simulink model "ES200A_CurrMeas"  (R2013b)
settings: Solver=FixedStepDiscrete  SolverMode=SingleTasking  StartTime=0.0  StopTime=1  FixedStep=0.000125  RelTol=1e-3
values from neighbouring files (symbols this model uses):
  ARCHGLBPRM_2PI_ULS_F32 = DataDict.Constant    [ES200A_CurrMeas_DataDict.m]
  CurrMeasEolGainMax = DataDict.Calibration    [ES200A_CurrMeas_DataDict.m]
  CurrMeasEolGainMin = DataDict.Calibration    [ES200A_CurrMeas_DataDict.m]
  CurrMeasEolGainNrOfSample = DataDict.Calibration    [ES200A_CurrMeas_DataDict.m]
  CurrMeasEolGainNumer = DataDict.Calibration    [ES200A_CurrMeas_DataDict.m]
  CurrMeasEolMaxMotVel = DataDict.Calibration    [ES200A_CurrMeas_DataDict.m]
  CurrMeasEolOffsHiBrdgVltgMin = DataDict.Calibration    [ES200A_CurrMeas_DataDict.m]
  CurrMeasEolOffsHiCmuOffs = DataDict.Calibration    [ES200A_CurrMeas_DataDict.m]
  CurrMeasEolOffsLoCmuOffs = DataDict.Calibration    [ES200A_CurrMeas_DataDict.m]
  CurrMeasEolOffsMax = DataDict.Calibration    [ES200A_CurrMeas_DataDict.m]
  CurrMeasEolOffsMin = DataDict.Calibration    [ES200A_CurrMeas_DataDict.m]
  CurrMeasEolOffsNrOfSample = DataDict.Calibration    [ES200A_CurrMeas_DataDict.m]
  CurrMeasEolTranCntrThd = DataDict.Calibration    [ES200A_CurrMeas_DataDict.m]
  CurrMeasMinRqrdPhaOnTi = DataDict.Calibration    [ES200A_CurrMeas_DataDict.m]
  CurrMeasMotAgCompuDly = DataDict.Calibration    [ES200A_CurrMeas_DataDict.m]
  CurrMeasMotCurrAdcVlyWrmIninMax = DataDict.Calibration    [ES200A_CurrMeas_DataDict.m]
  CurrMeasMotCurrAdcVlyWrmIninMin = DataDict.Calibration    [ES200A_CurrMeas_DataDict.m]
  CurrMeasNtc0x05DFailStep = DataDict.Calibration    [ES200A_CurrMeas_DataDict.m]
  CurrMeasNtc0x05DPassStep = DataDict.Calibration    [ES200A_CurrMeas_DataDict.m]
  CurrMeasNtc0x06DFailStep = DataDict.Calibration    [ES200A_CurrMeas_DataDict.m]
  CurrMeasNtc0x06DPassStep = DataDict.Calibration    [ES200A_CurrMeas_DataDict.m]
  DEGREES30_MOTRAD_F32 = DataDict.Constant    [ES200A_CurrMeas_DataDict.m]
  DIFOFFSRNGCHKMAX_VOLT_F32 = DataDict.Constant    [ES200A_CurrMeas_DataDict.m]
  ELECGLBPRM_IVTRCNT_CNT_U08 = DataDict.ConfigParam    [ES200A_CurrMeas_DataDict.m]
  ELECGLBPRM_STRTUPSTCURRMEASWRMININTESTSTRT_CNT_U08 = DataDict.Constant    [ES200A_CurrMeas_DataDict.m]
  FLTINJ_CURRMEAS_MOTCURRCORRDA = DataDict.Constant    [ES200A_CurrMeas_DataDict.m]
  FLTINJ_CURRMEAS_MOTCURRCORRDD = DataDict.Constant    [ES200A_CurrMeas_DataDict.m]
  FLTINJ_CURRMEAS_TESTOK = DataDict.Constant    [ES200A_CurrMeas_DataDict.m]
  MAXCURRCORRD_AMPR_F32 = DataDict.Constant    [ES200A_CurrMeas_DataDict.m]
  PhaABCMeasdOutOfRng = DataDict.NTC    [ES200A_CurrMeas_DataDict.m]
  PhaDEFMeasOutOfRng = DataDict.NTC    [ES200A_CurrMeas_DataDict.m]
  SysGlbPrmMotPoleCnt = DataDict.ImprtdCal    [ES200A_CurrMeas_DataDict.m]
libraries: simulink x10, FixdToFloat x1
(part 6 of 7)

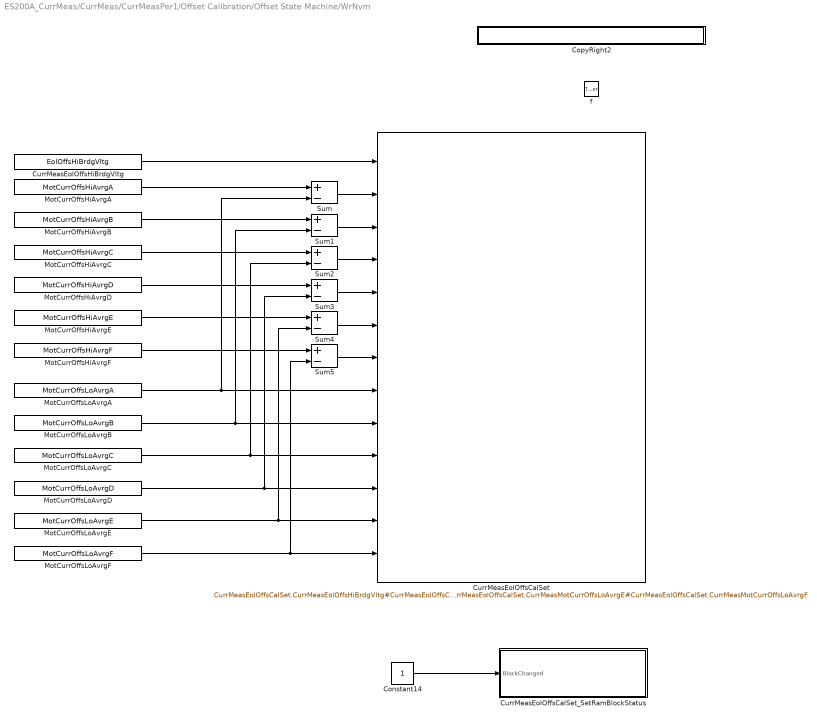
== system ES200A_CurrMeas/CurrMeas/CurrMeasPer1/Offset Calibration/Offset State Machine/WrNvm ==
  f : TriggerPort  TriggerType=function-call
      settings: CopyFcn=Stateflow.SLINSF.SimulinkMan.removeBlockPreDeleteFcn  PreDeleteFcn=Stateflow.SLINSF.SimulinkMan.unsafePredeleteFcn
  Constant14 : Constant  OutDataTypeStr=single
  CopyRight2 : Subsystem  Description=|  mask(Copyright Information){none=on}
      | Copyright info block.                                               
      |                                                                     
      | Place copyright information at the top of every subsystem in design.
      mask prompts: none "No parameters"
      mask help: Place copyright information at the top of every subsystem in design.
      mask Display:
      | NxtrConf = 'Nexteer Confidential';
      | 
      | sys = bdroot; %handle for the current model ("system")
      | first = get_param(sys,'Created');
      | first = first(end-3:end);  %year is last four digits
      | 
      | last = get_param(sys,'LastModifiedDate');
      | if isempty(last)
      |     last = datestr(now,'yyyy');
      | else
      |     last = last(end-3:end);
      | end
      | 
      | if strcmp(first,last)
      |     fprintf('%s -- Copyright %s Nexteer',NxtrConf,first)
      | else
      |     fprintf('%s -- %s%s- %s Nexteer',NxtrConf,char(169),first,last)
      | end
  CurrMeasEolOffsCalSet : DataStoreWrite  RequirementInfo={'linktype_rmi_doors' '000089bc (/ESG Group/FDD Module Requirements/EA4 Specific/ES200A_CurrMeas)' '#ES200A_138' 'true' 'REQ: ES200A_138' '' } %GIDa_9629138e_22c6_4a2f_a212_b03a049f0344  DataStoreName=CurrMeasEolOffsCalSet  DataStoreElements=CurrMeasEolOffsCalSet.CurrMeasEolOffsHiBrdgVltg#CurrMeasEolOffsCalSet.CurrMeasMotCurrEolOffsDifA#CurrMeasEolOffsCalSet.CurrMeasMotCurrEolOffsDifB#CurrMeasEolOffsCalSet.CurrMeasMotCurrEolOffsDifC#CurrMeasEolOffsCalSet.CurrMeasMotCurrEolOffsDifD#CurrMeasEolOffsCalSet.CurrMeasMotCurrEolOffsDifE#CurrMeasEolOffsCalSet.CurrMeasMotCurrEolOffsDifF#CurrMeasEolOffsCalSet.CurrMeasMotCurrOffsLoAvrgA#CurrMeasEolOffsCalSet.CurrMeasMotCurrOffsLoAvrgB#CurrMeasEolOffsCalSet.CurrMeasMotCurrOffsLoAvrgC#CurrMeasEolOffsCalSet.CurrMeasMotCurrOffsLoAvrgD#CurrMeasEolOffsCalSet.CurrMeasMotCurrOffsLoAvrgE#CurrMeasEolOffsCalSet.CurrMeasMotCurrOffsLoAvrgF
  CurrMeasEolOffsCalSet_SetRamBlockStatus : Subsystem  RequirementInfo={'linktype_rmi_doors' '000089bc (/ESG Group/FDD Module Requirements/EA4 Specific/ES200A_CurrMeas)' '#ES200A_138' 'true' 'REQ: ES200A_138' '' } %GIDa_8abdf95c_ca53_47b3_a6c5_ea06d33b5ee8  TreatAsAtomicUnit=on
  CurrMeasEolOffsHiBrdgVltg : DataStoreRead  DataStoreName=EolOffsHiBrdgVltg  DataStoreElements=EolOffsHiBrdgVltg
  MotCurrOffsHiAvrgA : DataStoreRead  DataStoreName=MotCurrOffsHiAvrgA  DataStoreElements=MotCurrOffsHiAvrgA
  MotCurrOffsHiAvrgB : DataStoreRead  DataStoreName=MotCurrOffsHiAvrgB  DataStoreElements=MotCurrOffsHiAvrgB
  MotCurrOffsHiAvrgC : DataStoreRead  DataStoreName=MotCurrOffsHiAvrgC  DataStoreElements=MotCurrOffsHiAvrgC
  MotCurrOffsHiAvrgD : DataStoreRead  DataStoreName=MotCurrOffsHiAvrgD  DataStoreElements=MotCurrOffsHiAvrgD
  MotCurrOffsHiAvrgE : DataStoreRead  DataStoreName=MotCurrOffsHiAvrgE  DataStoreElements=MotCurrOffsHiAvrgE
  MotCurrOffsHiAvrgF : DataStoreRead  DataStoreName=MotCurrOffsHiAvrgF  DataStoreElements=MotCurrOffsHiAvrgF
  MotCurrOffsLoAvrgA : DataStoreRead  DataStoreName=MotCurrOffsLoAvrgA  DataStoreElements=MotCurrOffsLoAvrgA
  MotCurrOffsLoAvrgB : DataStoreRead  DataStoreName=MotCurrOffsLoAvrgB  DataStoreElements=MotCurrOffsLoAvrgB
  MotCurrOffsLoAvrgC : DataStoreRead  DataStoreName=MotCurrOffsLoAvrgC  DataStoreElements=MotCurrOffsLoAvrgC
  MotCurrOffsLoAvrgD : DataStoreRead  DataStoreName=MotCurrOffsLoAvrgD  DataStoreElements=MotCurrOffsLoAvrgD
  MotCurrOffsLoAvrgE : DataStoreRead  DataStoreName=MotCurrOffsLoAvrgE  DataStoreElements=MotCurrOffsLoAvrgE
  MotCurrOffsLoAvrgF : DataStoreRead  DataStoreName=MotCurrOffsLoAvrgF  DataStoreElements=MotCurrOffsLoAvrgF
  Sum{,1..5} (6 alike) : Sum  Inputs=+-
  wires:
  CurrMeasEolOffsHiBrdgVltg/1 -> CurrMeasEolOffsCalSet/1
  Sum/1 -> CurrMeasEolOffsCalSet/2
  Sum1/1 -> CurrMeasEolOffsCalSet/3
  Sum2/1 -> CurrMeasEolOffsCalSet/4
  Sum3/1 -> CurrMeasEolOffsCalSet/5
  Sum4/1 -> CurrMeasEolOffsCalSet/6
  Sum5/1 -> CurrMeasEolOffsCalSet/7
  MotCurrOffsLoAvrgC/1 -> Sum2/2, CurrMeasEolOffsCalSet/10
  MotCurrOffsLoAvrgB/1 -> Sum1/2, CurrMeasEolOffsCalSet/9
  MotCurrOffsLoAvrgD/1 -> Sum3/2, CurrMeasEolOffsCalSet/11
  MotCurrOffsLoAvrgE/1 -> Sum4/2, CurrMeasEolOffsCalSet/12
  MotCurrOffsLoAvrgA/1 -> Sum/2, CurrMeasEolOffsCalSet/8
  MotCurrOffsLoAvrgF/1 -> CurrMeasEolOffsCalSet/13, Sum5/2
  Constant14/1 -> CurrMeasEolOffsCalSet_SetRamBlockStatus/1("BlockChanged ")
  MotCurrOffsHiAvrgA/1 -> Sum/1
  MotCurrOffsHiAvrgB/1 -> Sum1/1
  MotCurrOffsHiAvrgC/1 -> Sum2/1
  MotCurrOffsHiAvrgD/1 -> Sum3/1
  MotCurrOffsHiAvrgE/1 -> Sum4/1
  MotCurrOffsHiAvrgF/1 -> Sum5/1

== system ES200A_CurrMeas/CurrMeas/CurrMeasPer2/Chart1/CalcMotCurrMotAgCorrd/+//- 2*Pi Rollover ==
  MotAgCorrdRaw : Inport
  -2*pi Rollover : Subsystem  TreatAsAtomicUnit=on
  2*pi Rollover : Subsystem  TreatAsAtomicUnit=on
  Constant : Constant  Value=-1  OutDataTypeStr=single
  Constant1 : Constant  Value=ARCHGLBPRM_2PI_ULS_F32  OutDataTypeStr=Inherit: Inherit via back propagation
  Constant4 : Constant  Value=ARCHGLBPRM_2PI_ULS_F32  OutDataTypeStr=Inherit: Inherit via back propagation
  CopyRight2 : Subsystem  Description=|  mask(Copyright Information){none=on}
      | Copyright info block.                                               
      |                                                                     
      | Place copyright information at the top of every subsystem in design.
      mask prompts: none "No parameters"
      mask help: Place copyright information at the top of every subsystem in design.
      mask Display:
      | NxtrConf = 'Nexteer Confidential';
      | 
      | sys = bdroot; %handle for the current model ("system")
      | first = get_param(sys,'Created');
      | first = first(end-3:end);  %year is last four digits
      | 
      | last = get_param(sys,'LastModifiedDate');
      | if isempty(last)
      |     last = datestr(now,'yyyy');
      | else
      |     last = last(end-3:end);
      | end
      | 
      | if strcmp(first,last)
      |     fprintf('%s -- Copyright %s Nexteer',NxtrConf,first)
      | else
      |     fprintf('%s -- %s%s- %s Nexteer',NxtrConf,char(169),first,last)
      | end
  If : If  NumInputs=3  IfExpression=u1 > u2  ElseIfExpressions=u1 < u3
  Merge : Merge  Inputs=3
  Pass Through : Subsystem  TreatAsAtomicUnit=on
  Product : Product
  MotCtrlCurrMeasMotAgCorrd : Outport
  wires:
  If/2 -> -2*pi Rollover/Action
  MotAgCorrdRaw/1 -> If/1, [MotAgCorrdRaw]
  Constant4/1 -> If/2
  Constant1/1 -> Product/1
  If/1 -> 2*pi Rollover/Action
  [MotAgCorrdRaw] -> 2*pi Rollover/1(MotAgCorrdRaw)
  [MotAgCorrdRaw] -> -2*pi Rollover/1(MotAgCorrdRaw)
  If/3 -> Pass Through/Action
  2*pi Rollover/1(Out1) -> Merge/1
  -2*pi Rollover/1(Out1) -> Merge/2
  Pass Through/1(Out1) -> Merge/3
  [MotAgCorrdRaw] -> Pass Through/1(MotAgCorrdRaw)
  Merge/1 -> MotCtrlCurrMeasMotAgCorrd/1
  Constant/1 -> Product/2
  Product/1 -> If/3

== system ES200A_CurrMeas/CurrMeas/CurrMeasPer2/Chart1/CalcMotCurrMotAgCorrd/CopyRight2 ==

== system ES200A_CurrMeas/CurrMeas/CurrMeasPer2/Chart1/OffsCalcABC/CopyRight2 ==

== system ES200A_CurrMeas/CurrMeas/CurrMeasPer2/Chart1/OffsCalcDEF/CopyRight2 ==

== system ES200A_CurrMeas/CurrMeas/CurrMeasPer2/Chart1/ProtocolChkENABC/CopyRight2 ==

== system ES200A_CurrMeas/CurrMeas/CurrMeasPer2/Chart1/ProtocolChkENABC/FltInj_u08 ==
  note: This block requires no modification by FDD author.
      |
      | This block does not actually simulate any fault injection.  It is simply a pass-thru.
      |
      | The Constant port (#2) simply terminates its signal, but we are trying to force the FDD author
      | to properly use the FltInjectionLocType enumeration in FDD model.
  note: EA4.x Fault Injection
  Signal_In : Inport
  Constant : Inport  Port=2
  CopyRight2 : Subsystem  Description=|  mask(Copyright Information){none=on}
      | Copyright info block.                                               
      |                                                                     
      | Place copyright information at the top of every subsystem in design.
      mask prompts: none "No parameters"
      mask help: Place copyright information at the top of every subsystem in design.
      mask Display:
      | NxtrConf = 'Nexteer Confidential';
      | 
      | sys = bdroot; %handle for the current model ("system")
      | first = get_param(sys,'Created');
      | first = first(end-3:end);  %year is last four digits
      | 
      | last = get_param(sys,'LastModifiedDate');
      | if isempty(last)
      |     last = datestr(now,'yyyy');
      | else
      |     last = last(end-3:end);
      | end
      | 
      | if strcmp(first,last)
      |     fprintf('%s -- Copyright %s Nexteer',NxtrConf,first)
      | else
      |     fprintf('%s -- %s%s- %s Nexteer',NxtrConf,char(169),first,last)
      | end
  Terminator : Terminator
  Signal_Out : Outport
  wires:
  Signal_In/1 -> Signal_Out/1
  Constant/1 -> Terminator/1

== system ES200A_CurrMeas/CurrMeas/CurrMeasPer2/Chart1/ProtocolChkENDEF/CopyRight2 ==

== system ES200A_CurrMeas/CurrMeas/CurrMeasPer2/FltInj_f32/CopyRight2 ==

== system ES200A_CurrMeas/CurrMeas/CurrMeasPer3/Chart1/GetNtc5DQlfrSts/CopyRight2 ==

== system ES200A_CurrMeas/CurrMeas/CurrMeasPer3/Chart1/GetNtc5DQlfrSts/GetNtcQlfrSts ==
  NtcNr : Inport
  CopyRight2 : Subsystem  Description=|  mask(Copyright Information){none=on}
      | Copyright info block.                                               
      |                                                                     
      | Place copyright information at the top of every subsystem in design.
      mask prompts: none "No parameters"
      mask help: Place copyright information at the top of every subsystem in design.
      mask Display:
      | NxtrConf = 'Nexteer Confidential';
      | 
      | sys = bdroot; %handle for the current model ("system")
      | first = get_param(sys,'Created');
      | first = first(end-3:end);  %year is last four digits
      | 
      | last = get_param(sys,'LastModifiedDate');
      | if isempty(last)
      |     last = datestr(now,'yyyy');
      | else
      |     last = last(end-3:end);
      | end
      | 
      | if strcmp(first,last)
      |     fprintf('%s -- Copyright %s Nexteer',NxtrConf,first)
      | else
      |     fprintf('%s -- %s%s- %s Nexteer',NxtrConf,char(169),first,last)
      | end
  Data Store Read1 : DataStoreRead  DataStoreName=NtcQlfr5D
  Terminator1 : Terminator
  NtcQlfr : Outport
  wires:
  NtcNr/1 -> Terminator1/1
  Data Store Read1/1 -> NtcQlfr/1

== system ES200A_CurrMeas/CurrMeas/CurrMeasPer3/Chart1/GetNtc6DQlfrSts/CopyRight2 ==

== system ES200A_CurrMeas/CurrMeas/CurrMeasPer3/Chart1/GetNtc6DQlfrSts/GetNtcQlfrSts ==
  NtcNr : Inport
  CopyRight2 : Subsystem  Description=|  mask(Copyright Information){none=on}
      | Copyright info block.                                               
      |                                                                     
      | Place copyright information at the top of every subsystem in design.
      mask prompts: none "No parameters"
      mask help: Place copyright information at the top of every subsystem in design.
      mask Display:
      | NxtrConf = 'Nexteer Confidential';
      | 
      | sys = bdroot; %handle for the current model ("system")
      | first = get_param(sys,'Created');
      | first = first(end-3:end);  %year is last four digits
      | 
      | last = get_param(sys,'LastModifiedDate');
      | if isempty(last)
      |     last = datestr(now,'yyyy');
      | else
      |     last = last(end-3:end);
      | end
      | 
      | if strcmp(first,last)
      |     fprintf('%s -- Copyright %s Nexteer',NxtrConf,first)
      | else
      |     fprintf('%s -- %s%s- %s Nexteer',NxtrConf,char(169),first,last)
      | end
  Data Store Read2 : DataStoreRead  DataStoreName=NtcQlfr6D
  Terminator1 : Terminator
  NtcQlfr : Outport
  wires:
  NtcNr/1 -> Terminator1/1
  Data Store Read2/1 -> NtcQlfr/1

== system ES200A_CurrMeas/CurrMeas/CurrMeasPer3/Chart1/RangeChkWIABC/CopyRight2 ==

== system ES200A_CurrMeas/CurrMeas/CurrMeasPer3/Chart1/RangeChkWIABC/If Action Subsystem2 ==
  Action Port : ActionPort  ActionType=then
  Constant : Constant
  CopyRight2 : Subsystem  Description=|  mask(Copyright Information){none=on}
      | Copyright info block.                                               
      |                                                                     
      | Place copyright information at the top of every subsystem in design.
      mask prompts: none "No parameters"
      mask help: Place copyright information at the top of every subsystem in design.
      mask Display:
      | NxtrConf = 'Nexteer Confidential';
      | 
      | sys = bdroot; %handle for the current model ("system")
      | first = get_param(sys,'Created');
      | first = first(end-3:end);  %year is last four digits
      | 
      | last = get_param(sys,'LastModifiedDate');
      | if isempty(last)
      |     last = datestr(now,'yyyy');
      | else
      |     last = last(end-3:end);
      | end
      | 
      | if strcmp(first,last)
      |     fprintf('%s -- Copyright %s Nexteer',NxtrConf,first)
      | else
      |     fprintf('%s -- %s%s- %s Nexteer',NxtrConf,char(169),first,last)
      | end
  Out1 : Outport
  wires:
  Constant/1 -> Out1/1

== system ES200A_CurrMeas/CurrMeas/CurrMeasPer3/Chart1/RangeChkWIABC/If Action Subsystem3 ==
  Action Port : ActionPort  ActionType=else
  Constant : Constant  Value=0
  CopyRight2 : Subsystem  Description=|  mask(Copyright Information){none=on}
      | Copyright info block.                                               
      |                                                                     
      | Place copyright information at the top of every subsystem in design.
      mask prompts: none "No parameters"
      mask help: Place copyright information at the top of every subsystem in design.
      mask Display:
      | NxtrConf = 'Nexteer Confidential';
      | 
      | sys = bdroot; %handle for the current model ("system")
      | first = get_param(sys,'Created');
      | first = first(end-3:end);  %year is last four digits
      | 
      | last = get_param(sys,'LastModifiedDate');
      | if isempty(last)
      |     last = datestr(now,'yyyy');
      | else
      |     last = last(end-3:end);
      | end
      | 
      | if strcmp(first,last)
      |     fprintf('%s -- Copyright %s Nexteer',NxtrConf,first)
      | else
      |     fprintf('%s -- %s%s- %s Nexteer',NxtrConf,char(169),first,last)
      | end
  Out1 : Outport
  wires:
  Constant/1 -> Out1/1

== system ES200A_CurrMeas/CurrMeas/CurrMeasPer3/Chart1/RangeChkWIDEF/CopyRight2 ==

== system ES200A_CurrMeas/CurrMeas/CurrMeasPer3/Chart1/RangeChkWIDEF/If Action Subsystem2 ==
  Action Port : ActionPort  ActionType=then
  Constant : Constant
  CopyRight2 : Subsystem  Description=|  mask(Copyright Information){none=on}
      | Copyright info block.                                               
      |                                                                     
      | Place copyright information at the top of every subsystem in design.
      mask prompts: none "No parameters"
      mask help: Place copyright information at the top of every subsystem in design.
      mask Display:
      | NxtrConf = 'Nexteer Confidential';
      | 
      | sys = bdroot; %handle for the current model ("system")
      | first = get_param(sys,'Created');
      | first = first(end-3:end);  %year is last four digits
      | 
      | last = get_param(sys,'LastModifiedDate');
      | if isempty(last)
      |     last = datestr(now,'yyyy');
      | else
      |     last = last(end-3:end);
      | end
      | 
      | if strcmp(first,last)
      |     fprintf('%s -- Copyright %s Nexteer',NxtrConf,first)
      | else
      |     fprintf('%s -- %s%s- %s Nexteer',NxtrConf,char(169),first,last)
      | end
  Out1 : Outport
  wires:
  Constant/1 -> Out1/1

== system ES200A_CurrMeas/CurrMeas/CurrMeasPer3/Chart1/RangeChkWIDEF/If Action Subsystem3 ==
  Action Port : ActionPort  ActionType=else
  Constant : Constant  Value=0
  CopyRight2 : Subsystem  Description=|  mask(Copyright Information){none=on}
      | Copyright info block.                                               
      |                                                                     
      | Place copyright information at the top of every subsystem in design.
      mask prompts: none "No parameters"
      mask help: Place copyright information at the top of every subsystem in design.
      mask Display:
      | NxtrConf = 'Nexteer Confidential';
      | 
      | sys = bdroot; %handle for the current model ("system")
      | first = get_param(sys,'Created');
      | first = first(end-3:end);  %year is last four digits
      | 
      | last = get_param(sys,'LastModifiedDate');
      | if isempty(last)
      |     last = datestr(now,'yyyy');
      | else
      |     last = last(end-3:end);
      | end
      | 
      | if strcmp(first,last)
      |     fprintf('%s -- Copyright %s Nexteer',NxtrConf,first)
      | else
      |     fprintf('%s -- %s%s- %s Nexteer',NxtrConf,char(169),first,last)
      | end
  Out1 : Outport
  wires:
  Constant/1 -> Out1/1

== system ES200A_CurrMeas/CurrMeas/CurrMeasPer3/Chart1/SetNtc5DSts/CopyRight2 ==

== system ES200A_CurrMeas/CurrMeas/CurrMeasPer3/Chart1/SetNtc5DSts/SetNtcSts ==
  note: Note:
      |
      | - "ISO Fault Debounce Design" Simulink block intent to use here for Simulation purpose only. Do not Code this block
  note: 1. Moved condition Action {ErrAcc = 0;
      | Qualifier =0;
      | } from 2nd Transition action to first trnasition action as there is no condition action in first transition action
      | Also changed SvcClr to 1
  NtcNr : Inport
  NtcStInfo : Inport  Port=2
  NtcSts : Inport  Port=3
  DebStep : Inport  Port=4
  CopyRight2 : Subsystem  Description=|  mask(Copyright Information){none=on}
      | Copyright info block.                                               
      |                                                                     
      | Place copyright information at the top of every subsystem in design.
      mask prompts: none "No parameters"
      mask help: Place copyright information at the top of every subsystem in design.
      mask Display:
      | NxtrConf = 'Nexteer Confidential';
      | 
      | sys = bdroot; %handle for the current model ("system")
      | first = get_param(sys,'Created');
      | first = first(end-3:end);  %year is last four digits
      | 
      | last = get_param(sys,'LastModifiedDate');
      | if isempty(last)
      |     last = datestr(now,'yyyy');
      | else
      |     last = last(end-3:end);
      | end
      | 
      | if strcmp(first,last)
      |     fprintf('%s -- Copyright %s Nexteer',NxtrConf,first)
      | else
      |     fprintf('%s -- %s%s- %s Nexteer',NxtrConf,char(169),first,last)
      | end
  Data Store Write : DataStoreWrite  DataStoreName=NtcQlfr5D
  Ground : Ground
  ISO Fault Debounce Design : Stateflow chart  TreatAsAtomicUnit=on
      settings: AttributesFormatString=|
      | Simulation Purpose Only.
      | Do Not Code this block
      | Diagnostic Manager Owns this requirement
  Scope1 : Scope  NumInputPorts=3
      settings: YMin=2~16384~-5  YMax=2~16384~5  SaveName=ScopeData5
  Terminator : Terminator
  Terminator1 : Terminator
  wires:
  NtcStInfo/1 -> Terminator1/1
  NtcNr/1 -> Terminator/1
  NtcSts/1 -> ISO Fault Debounce Design/1(NtcSts), Scope1/1
  DebStep/1 -> ISO Fault Debounce Design/2(DebStep), Scope1/2
  ISO Fault Debounce Design/1(Qualifier) -> Data Store Write/1, Scope1/3
  Ground/1 -> ISO Fault Debounce Design/3(SvcClr)

== system ES200A_CurrMeas/CurrMeas/CurrMeasPer3/Chart1/SetNtc6DSts/CopyRight2 ==

== system ES200A_CurrMeas/CurrMeas/CurrMeasPer3/Chart1/SetNtc6DSts/SetNtcSts ==
  note: Note:
      |
      | - "ISO Fault Debounce Design" Simulink block intent to use here for Simulation purpose only. Do not Code this block
  note: Moved condition Action {ErrAcc = 0;
      | Qualifier =0;
      | } from 2nd Transition action to first trnasition action as there is no condition action in first transition action
      | Also changed SvcClr to 1
  NtcNr : Inport
  NtcStInfo : Inport  Port=2
  NtcSts : Inport  Port=3
  DebStep : Inport  Port=4
  CopyRight2 : Subsystem  Description=|  mask(Copyright Information){none=on}
      | Copyright info block.                                               
      |                                                                     
      | Place copyright information at the top of every subsystem in design.
      mask prompts: none "No parameters"
      mask help: Place copyright information at the top of every subsystem in design.
      mask Display:
      | NxtrConf = 'Nexteer Confidential';
      | 
      | sys = bdroot; %handle for the current model ("system")
      | first = get_param(sys,'Created');
      | first = first(end-3:end);  %year is last four digits
      | 
      | last = get_param(sys,'LastModifiedDate');
      | if isempty(last)
      |     last = datestr(now,'yyyy');
      | else
      |     last = last(end-3:end);
      | end
      | 
      | if strcmp(first,last)
      |     fprintf('%s -- Copyright %s Nexteer',NxtrConf,first)
      | else
      |     fprintf('%s -- %s%s- %s Nexteer',NxtrConf,char(169),first,last)
      | end
  Data Store Write : DataStoreWrite  DataStoreName=NtcQlfr6D
  Ground : Ground
  ISO Fault Debounce Design : Stateflow chart  TreatAsAtomicUnit=on
      settings: AttributesFormatString=|
      | Simulation Purpose Only.
      | Do Not Code this block
      | Diagnostic Manager Owns this requirement
  Scope1 : Scope  NumInputPorts=3
      settings: YMin=-5~-5~-5  YMax=5~5~5  SaveName=ScopeData5
  Terminator : Terminator
  Terminator1 : Terminator
  wires:
  NtcStInfo/1 -> Terminator1/1
  NtcNr/1 -> Terminator/1
  NtcSts/1 -> ISO Fault Debounce Design/1(NtcSts), Scope1/1
  DebStep/1 -> ISO Fault Debounce Design/2(DebStep), Scope1/2
  ISO Fault Debounce Design/1(Qualifier) -> Data Store Write/1, Scope1/3
  Ground/1 -> ISO Fault Debounce Design/3(SvcClr)

== system ES200A_CurrMeas/CurrMeas/CurrMeasGainWrReq/IF/CurrMeasEolGainCalSet_SetRamBlockStatus/CopyRight2 ==

== system ES200A_CurrMeas/CurrMeas/CurrMeasOffsWrReq/IF/CurrMeasEolOffsCalSet_SetRamBlockStatus/CopyRight2 ==

== system ES200A_CurrMeas/CurrMeas/CurrMeasPer1/Gain Calibration/GainStateMachine/SetNtcSts/CopyRight2 ==

== system ES200A_CurrMeas/CurrMeas/CurrMeasPer1/Gain Calibration/GainStateMachine/SetNtcSts/SetNtcSts ==
  note: Note:
      |
      | - "ISO Fault Debounce Design" Simulink block intent to use here for Simulation purpose only. Do not Code this block
  NtcNr : Inport
  NtcStInfo : Inport  Port=2
  NtcSts : Inport  Port=3
  DebStep : Inport  Port=4
  CopyRight2 : Subsystem  Description=|  mask(Copyright Information){none=on}
      | Copyright info block.                                               
      |                                                                     
      | Place copyright information at the top of every subsystem in design.
      mask prompts: none "No parameters"
      mask help: Place copyright information at the top of every subsystem in design.
      mask Display:
      | NxtrConf = 'Nexteer Confidential';
      | 
      | sys = bdroot; %handle for the current model ("system")
      | first = get_param(sys,'Created');
      | first = first(end-3:end);  %year is last four digits
      | 
      | last = get_param(sys,'LastModifiedDate');
      | if isempty(last)
      |     last = datestr(now,'yyyy');
      | else
      |     last = last(end-3:end);
      | end
      | 
      | if strcmp(first,last)
      |     fprintf('%s -- Copyright %s Nexteer',NxtrConf,first)
      | else
      |     fprintf('%s -- %s%s- %s Nexteer',NxtrConf,char(169),first,last)
      | end
  Data Store Write : DataStoreWrite  DataStoreName=NtcQlfr1ED
  Ground : Ground
  ISO Fault Debounce Design : Stateflow chart  TreatAsAtomicUnit=on
      settings: AttributesFormatString=|
      | Simulation Purpose Only.
      | Do Not Code this block
      | Diagnostic Manager Owns this requirement
  Scope1 : Scope  NumInputPorts=3
      settings: YMin=-5~-5~-5  YMax=5~5~5  SaveName=ScopeData4
  Terminator : Terminator
  Terminator1 : Terminator
  wires:
  NtcStInfo/1 -> Terminator1/1
  NtcNr/1 -> Terminator/1
  NtcSts/1 -> ISO Fault Debounce Design/1(NtcSts), Scope1/1
  DebStep/1 -> ISO Fault Debounce Design/2(DebStep), Scope1/2
  ISO Fault Debounce Design/1(Qualifier) -> Scope1/3, Data Store Write/1  "Qualifier"
  Ground/1 -> ISO Fault Debounce Design/3(SvcClr)

== system ES200A_CurrMeas/CurrMeas/CurrMeasPer1/Gain Calibration/GainStateMachine/WrNvm/CopyRight2 ==

== system ES200A_CurrMeas/CurrMeas/CurrMeasPer1/Gain Calibration/GainStateMachine/WrNvm/CurrMeasEolGainCalSet_SetRamBlockStatus ==
  "BlockChanged " : Inport  RequirementInfo={} %GIDa_e825a47e_fdb5_416f_b5f2_d196e0b30ed6  OutDataTypeStr=single
  CopyRight2 : Subsystem  Description=|  mask(Copyright Information){none=on}
      | Copyright info block.                                               
      |                                                                     
      | Place copyright information at the top of every subsystem in design.
      mask prompts: none "No parameters"
      mask help: Place copyright information at the top of every subsystem in design.
      mask Display:
      | NxtrConf = 'Nexteer Confidential';
      | 
      | sys = bdroot; %handle for the current model ("system")
      | first = get_param(sys,'Created');
      | first = first(end-3:end);  %year is last four digits
      | 
      | last = get_param(sys,'LastModifiedDate');
      | if isempty(last)
      |     last = datestr(now,'yyyy');
      | else
      |     last = last(end-3:end);
      | end
      | 
      | if strcmp(first,last)
      |     fprintf('%s -- Copyright %s Nexteer',NxtrConf,first)
      | else
      |     fprintf('%s -- %s%s- %s Nexteer',NxtrConf,char(169),first,last)
      | end
  Terminator9 : Terminator
  wires:
  "BlockChanged "/1 -> Terminator9/1

== system ES200A_CurrMeas/CurrMeas/CurrMeasPer1/Offset Calibration/Offset State Machine/SetNtcSts/CopyRight2 ==

== system ES200A_CurrMeas/CurrMeas/CurrMeasPer1/Offset Calibration/Offset State Machine/SetNtcSts/SetNtcSts ==
  note: Note:
      |
      | - "ISO Fault Debounce Design" Simulink block intent to use here for Simulation purpose only. Do not Code this block
  NtcNr : Inport
  NtcStInfo : Inport  Port=2
  NtcSts : Inport  Port=3
  DebStep : Inport  Port=4
  CopyRight2 : Subsystem  Description=|  mask(Copyright Information){none=on}
      | Copyright info block.                                               
      |                                                                     
      | Place copyright information at the top of every subsystem in design.
      mask prompts: none "No parameters"
      mask help: Place copyright information at the top of every subsystem in design.
      mask Display:
      | NxtrConf = 'Nexteer Confidential';
      | 
      | sys = bdroot; %handle for the current model ("system")
      | first = get_param(sys,'Created');
      | first = first(end-3:end);  %year is last four digits
      | 
      | last = get_param(sys,'LastModifiedDate');
      | if isempty(last)
      |     last = datestr(now,'yyyy');
      | else
      |     last = last(end-3:end);
      | end
      | 
      | if strcmp(first,last)
      |     fprintf('%s -- Copyright %s Nexteer',NxtrConf,first)
      | else
      |     fprintf('%s -- %s%s- %s Nexteer',NxtrConf,char(169),first,last)
      | end
  Data Store Write : DataStoreWrite  DataStoreName=NtcQlfr1EC
  Ground : Ground
  ISO Fault Debounce Design : Stateflow chart  TreatAsAtomicUnit=on
      settings: AttributesFormatString=|
      | Simulation Purpose Only.
      | Do Not Code this block
      | Diagnostic Manager Owns this requirement
  Scope1 : Scope  NumInputPorts=3
      settings: YMin=-5~-5~-5  YMax=5~5~5  SaveName=ScopeData4
  Terminator : Terminator
  Terminator1 : Terminator
  wires:
  NtcStInfo/1 -> Terminator1/1
  NtcNr/1 -> Terminator/1
  NtcSts/1 -> ISO Fault Debounce Design/1(NtcSts), Scope1/1
  DebStep/1 -> ISO Fault Debounce Design/2(DebStep), Scope1/2
  ISO Fault Debounce Design/1(Qualifier) -> Scope1/3, Data Store Write/1  "Qualifier"
  Ground/1 -> ISO Fault Debounce Design/3(SvcClr)

== system ES200A_CurrMeas/CurrMeas/CurrMeasPer1/Offset Calibration/Offset State Machine/WrNvm/CopyRight2 ==

== system ES200A_CurrMeas/CurrMeas/CurrMeasPer1/Offset Calibration/Offset State Machine/WrNvm/CurrMeasEolOffsCalSet_SetRamBlockStatus ==
  "BlockChanged " : Inport  RequirementInfo={} %GIDa_ddbbad63_9bf8_4c81_98ef_dae72675538a  OutDataTypeStr=single
  CopyRight2 : Subsystem  Description=|  mask(Copyright Information){none=on}
      | Copyright info block.                                               
      |                                                                     
      | Place copyright information at the top of every subsystem in design.
      mask prompts: none "No parameters"
      mask help: Place copyright information at the top of every subsystem in design.
      mask Display:
      | NxtrConf = 'Nexteer Confidential';
      | 
      | sys = bdroot; %handle for the current model ("system")
      | first = get_param(sys,'Created');
      | first = first(end-3:end);  %year is last four digits
      | 
      | last = get_param(sys,'LastModifiedDate');
      | if isempty(last)
      |     last = datestr(now,'yyyy');
      | else
      |     last = last(end-3:end);
      | end
      | 
      | if strcmp(first,last)
      |     fprintf('%s -- Copyright %s Nexteer',NxtrConf,first)
      | else
      |     fprintf('%s -- %s%s- %s Nexteer',NxtrConf,char(169),first,last)
      | end
  Terminator9 : Terminator
  wires:
  "BlockChanged "/1 -> Terminator9/1

== system ES200A_CurrMeas/CurrMeas/CurrMeasPer2/Chart1/CalcMotCurrMotAgCorrd/+//- 2*Pi Rollover/-2*pi Rollover ==
  MotAgCorrdRaw : Inport
  Action Port : ActionPort  ActionType=elseif
  Add : Sum
  Constant4 : Constant  Value=ARCHGLBPRM_2PI_ULS_F32  OutDataTypeStr=Inherit: Inherit via back propagation
  CopyRight2 : Subsystem  Description=|  mask(Copyright Information){none=on}
      | Copyright info block.                                               
      |                                                                     
      | Place copyright information at the top of every subsystem in design.
      mask prompts: none "No parameters"
      mask help: Place copyright information at the top of every subsystem in design.
      mask Display:
      | NxtrConf = 'Nexteer Confidential';
      | 
      | sys = bdroot; %handle for the current model ("system")
      | first = get_param(sys,'Created');
      | first = first(end-3:end);  %year is last four digits
      | 
      | last = get_param(sys,'LastModifiedDate');
      | if isempty(last)
      |     last = datestr(now,'yyyy');
      | else
      |     last = last(end-3:end);
      | end
      | 
      | if strcmp(first,last)
      |     fprintf('%s -- Copyright %s Nexteer',NxtrConf,first)
      | else
      |     fprintf('%s -- %s%s- %s Nexteer',NxtrConf,char(169),first,last)
      | end
  Out1 : Outport
  wires:
  MotAgCorrdRaw/1 -> Add/1
  Constant4/1 -> Add/2
  Add/1 -> Out1/1

== system ES200A_CurrMeas/CurrMeas/CurrMeasPer2/Chart1/CalcMotCurrMotAgCorrd/+//- 2*Pi Rollover/2*pi Rollover ==
  MotAgCorrdRaw : Inport
  Action Port : ActionPort  ActionType=then
  Constant4 : Constant  Value=ARCHGLBPRM_2PI_ULS_F32  OutDataTypeStr=Inherit: Inherit via back propagation
  CopyRight2 : Subsystem  Description=|  mask(Copyright Information){none=on}
      | Copyright info block.                                               
      |                                                                     
      | Place copyright information at the top of every subsystem in design.
      mask prompts: none "No parameters"
      mask help: Place copyright information at the top of every subsystem in design.
      mask Display:
      | NxtrConf = 'Nexteer Confidential';
      | 
      | sys = bdroot; %handle for the current model ("system")
      | first = get_param(sys,'Created');
      | first = first(end-3:end);  %year is last four digits
      | 
      | last = get_param(sys,'LastModifiedDate');
      | if isempty(last)
      |     last = datestr(now,'yyyy');
      | else
      |     last = last(end-3:end);
      | end
      | 
      | if strcmp(first,last)
      |     fprintf('%s -- Copyright %s Nexteer',NxtrConf,first)
      | else
      |     fprintf('%s -- %s%s- %s Nexteer',NxtrConf,char(169),first,last)
      | end
  Subtract : Sum  Inputs=+-
  Out1 : Outport
  wires:
  MotAgCorrdRaw/1 -> Subtract/1
  Constant4/1 -> Subtract/2
  Subtract/1 -> Out1/1

== system ES200A_CurrMeas/CurrMeas/CurrMeasPer2/Chart1/CalcMotCurrMotAgCorrd/+//- 2*Pi Rollover/CopyRight2 ==

== system ES200A_CurrMeas/CurrMeas/CurrMeasPer2/Chart1/CalcMotCurrMotAgCorrd/+//- 2*Pi Rollover/Pass Through ==
  MotAgCorrdRaw : Inport
  Action Port : ActionPort  ActionType=else
  CopyRight2 : Subsystem  Description=|  mask(Copyright Information){none=on}
      | Copyright info block.                                               
      |                                                                     
      | Place copyright information at the top of every subsystem in design.
      mask prompts: none "No parameters"
      mask help: Place copyright information at the top of every subsystem in design.
      mask Display:
      | NxtrConf = 'Nexteer Confidential';
      | 
      | sys = bdroot; %handle for the current model ("system")
      | first = get_param(sys,'Created');
      | first = first(end-3:end);  %year is last four digits
      | 
      | last = get_param(sys,'LastModifiedDate');
      | if isempty(last)
      |     last = datestr(now,'yyyy');
      | else
      |     last = last(end-3:end);
      | end
      | 
      | if strcmp(first,last)
      |     fprintf('%s -- Copyright %s Nexteer',NxtrConf,first)
      | else
      |     fprintf('%s -- %s%s- %s Nexteer',NxtrConf,char(169),first,last)
      | end
  Out1 : Outport
  wires:
  MotAgCorrdRaw/1 -> Out1/1

== system ES200A_CurrMeas/CurrMeas/CurrMeasPer2/Chart1/ProtocolChkENABC/FltInj_u08/CopyRight2 ==

== system ES200A_CurrMeas/CurrMeas/CurrMeasPer3/Chart1/GetNtc5DQlfrSts/GetNtcQlfrSts/CopyRight2 ==

== system ES200A_CurrMeas/CurrMeas/CurrMeasPer3/Chart1/GetNtc6DQlfrSts/GetNtcQlfrSts/CopyRight2 ==

== system ES200A_CurrMeas/CurrMeas/CurrMeasPer3/Chart1/RangeChkWIABC/If Action Subsystem2/CopyRight2 ==

== system ES200A_CurrMeas/CurrMeas/CurrMeasPer3/Chart1/RangeChkWIABC/If Action Subsystem3/CopyRight2 ==

== system ES200A_CurrMeas/CurrMeas/CurrMeasPer3/Chart1/RangeChkWIDEF/If Action Subsystem2/CopyRight2 ==

== system ES200A_CurrMeas/CurrMeas/CurrMeasPer3/Chart1/RangeChkWIDEF/If Action Subsystem3/CopyRight2 ==

== system ES200A_CurrMeas/CurrMeas/CurrMeasPer3/Chart1/SetNtc5DSts/SetNtcSts/CopyRight2 ==

== system ES200A_CurrMeas/CurrMeas/CurrMeasPer3/Chart1/SetNtc6DSts/SetNtcSts/CopyRight2 ==

== system ES200A_CurrMeas/CurrMeas/CurrMeasPer1/Gain Calibration/GainStateMachine/SetNtcSts/SetNtcSts/CopyRight2 ==

== system ES200A_CurrMeas/CurrMeas/CurrMeasPer1/Gain Calibration/GainStateMachine/WrNvm/CurrMeasEolGainCalSet_SetRamBlockStatus/CopyRight2 ==

== system ES200A_CurrMeas/CurrMeas/CurrMeasPer1/Offset Calibration/Offset State Machine/SetNtcSts/SetNtcSts/CopyRight2 ==

== system ES200A_CurrMeas/CurrMeas/CurrMeasPer1/Offset Calibration/Offset State Machine/WrNvm/CurrMeasEolOffsCalSet_SetRamBlockStatus/CopyRight2 ==

== system ES200A_CurrMeas/CurrMeas/CurrMeasPer2/Chart1/CalcMotCurrMotAgCorrd/+//- 2*Pi Rollover/-2*pi Rollover/CopyRight2 ==

== system ES200A_CurrMeas/CurrMeas/CurrMeasPer2/Chart1/CalcMotCurrMotAgCorrd/+//- 2*Pi Rollover/2*pi Rollover/CopyRight2 ==

== system ES200A_CurrMeas/CurrMeas/CurrMeasPer2/Chart1/CalcMotCurrMotAgCorrd/+//- 2*Pi Rollover/Pass Through/CopyRight2 ==

== stateflow chart ES200A_CurrMeas/CurrMeas/CurrMeasPer3/Chart1/SetNtc6DSts/SetNtcSts/ISO Fault Debounce Design ==
  note: NTCSTS_PASSD           (0)
      | NTCSTS_FAILD             (1)
      | NTCSTS_PREPASSD   (2)
      | NTCSTS_PREFAILD     (3)
      |
      | SIGQLFR_NORES        (0)
      | SIGQLFR_PASSD         (1)
      | SIGQLFR_FAILD           (2)
  note: Pass Loop
  note: Fail Loop
  note: 
  note: Moved condition Action {ErrAcc = 0;
      | Qualifier =0;
      | } from 2nd Transition action to first trnasition action as there is no condition action in first transition action
      | Also changed SvcClr to 1
  (default) -> (junction 89)
  (junction 89) -> (junction 95) [order 1] : [NtcSts ==3]
  (junction 89) -> (junction 93) [order 2] : [NtcSts ==2]
  (junction 89) -> (junction 141) [order 3] : [NtcSts ==1]
      | { ErrAcc = 32767;
      | Qualifier =2;
      |  }
  (junction 89) -> (junction 141) [order 4] : [NtcSts ==0]
      | { ErrAcc = -32768;
      | Qualifier=1;
      | }
  (junction 95) -> (junction 103) [order 2]
  (junction 95) -> (junction 111) [order 1] : [ErrAcc <=0]
      | {ErrAcc = DebStep;}
  (junction 93) -> (junction 123) [order 2] : {
      | ErrAcc = ErrAcc - DebStep;
      | }
  (junction 93) -> (junction 123) [order 1] : [(ErrAcc - DebStep) <= -32768]
      | { ErrAcc = -32768;
      | Qualifier=1;
      | }
  (junction 103) -> (junction 111) [order 1] : [(ErrAcc + DebStep) <32767]
      | {ErrAcc = ErrAcc + DebStep;}
  (junction 103) -> (junction 111) [order 2] : {ErrAcc = 32767;
      | Qualifier =2;}
  (junction 123) -> (junction 141)
  (junction 111) -> (junction 141)
  (junction 141) -> (junction 159) [order 2]
  (junction 141) -> (junction 159) [order 1] : [SvcClr ==1]
      | {ErrAcc = 0;
      | Qualifier =0;
      | }
  data: NtcSts input uint8; Qualifier output uint8; DebStep input int32; ErrAcc local single; SvcClr input
